simulink model "Base_Map_S_P_L_cs"  (R2019a)
settings: Solver=FixedStepDiscrete  StartTime=0.0  StopTime=inf  FixedStep=1/300  RelTol=1e-3
PreLoadFcn:
  | mbxruntime.callbacks.PreLoadFcn(bdroot);
  | check_NUTS_defined
  | model_closed = 0;
  | assignin('base',['model_closed_' bdroot],false);
PostLoadFcn:
  | mbxruntime.callbacks.PostLoadFcn(bdroot);
InitFcn:
  | mbxruntime.callbacks.InitFcn(bdroot);
StartFcn:
  | mbxruntime.callbacks.StartFcn(bdroot);
StopFcn:
  | mbxruntime.callbacks.StopFcn(bdroot);;
  | 
model workspace: external: MAT-File .\Base_Map_S_P_L_cs_hws.mat (data not in the file)
undefined symbols (not defined in the file): DiscIntNeverNeededParam, Header, InitImageOutputDir, mbxruntime, Orientation, Pose, Poses, Poses_SL_Info, Position, tabledata
libraries: PBCSimulinkLibrary x53, simulink_extras x9, PreScanSimulinkLibrary x6, robotlib x6, PreScanUsefulBlocks x4, sharedtransform x3, aerolibutil x2, visionconversions x1, visionsinks x1
(part 5 of 7)

== system Base_Map_S_P_L_cs/Citroen_C3_Hatchback_1/Car_Pos_and_Orient ==
  In1 : Inport
  In2 : Inport  Port=2
  In3 : Inport  Port=3
  In4 : Inport  Port=4
  In5 : Inport  Port=5
  In6 : Inport  Port=6
  Data Type Conversion : DataTypeConversion
  Data Type Conversion1 : DataTypeConversion
  Data Type Conversion2 : DataTypeConversion
  Degrees to Radians1 : simulink_extras/Transformations/Degrees to Radians
  Degrees to Radians2 : simulink_extras/Transformations/Degrees to Radians
  Degrees to Radians5 : simulink_extras/Transformations/Degrees to Radians
  Mux : Mux
  Rotation Angles to Quaternions : sharedtransform/Rotation Angles to Quaternions  rotationOrder=XYZ  aMode=aMode
      settings: SourceProductName=Aerospace Blockset  SourceProductBaseCode=AE
  Vector Concatenate2 : Concatenate  NumInputs=3
  Out1 : Outport
  wires:
  Degrees to Radians1/1 -> Vector Concatenate2/2
  Degrees to Radians5/1 -> Vector Concatenate2/1
  Vector Concatenate2/1 -> Rotation Angles to Quaternions/1
  Degrees to Radians2/1 -> Vector Concatenate2/3
  In1/1 -> Data Type Conversion/1
  In2/1 -> Data Type Conversion1/1
  In3/1 -> Data Type Conversion2/1
  In4/1 -> Degrees to Radians5/1
  In5/1 -> Degrees to Radians1/1
  In6/1 -> Degrees to Radians2/1
  Data Type Conversion/1 -> Mux/1
  Data Type Conversion1/1 -> Mux/2
  Data Type Conversion2/1 -> Mux/3
  Rotation Angles to Quaternions/1 -> Mux/4
  Mux/1 -> Out1/1

== system Base_Map_S_P_L_cs/Citroen_C3_Hatchback_1/Dynamics_Empty ==
  note: For state mode 'Dynamic' positions
      | are not taken into account, as they
      | are computed by integrating velocity.
      | Click annotation for Help.
  Ground_{1..8} (8 alike) : Ground
  MuxState : Subsystem  Tag=mux/State  mask(Empty Dynamics State Block){positioningmode=on, TimeStep=1/300}
      mask prompts: positioningmode "Positioning Mode"; TimeStep "Auto Assigned: Time Step [s]"
      mask help:
      | Build the state of an actor based on user input.
      | The user can either use positioning mode or dynamics mode.
      | - When using positioning mode the position and orientation of the actor are set directly based on the input. Expected input is relative to the initial position and orientation of the actor. It's also possible to specify the velocity of the actor, though this input isn't used, only passed on.
      | - When using dynamics mode the position input is ignored. Expected input is velocity and orientation. The velocity is relative the current orientation of the actor, while orientation is relative to its initial orientation. The position of the actor is calculated based on the velocity and orientation given.
      settings: DeleteFcn=PreScanBlockDeleteFcn;
  STATE_Citroen_C3_Hatchback_1 : Subsystem  Tag=mux/StatePort  Priority=0  LoadFcn=load PrescanStateActuatorData  mask(PreScan Sink Block: State){x0=181.3426, y0=102.1129, z0=0.58, Roll0=0, Pitch0=0, Yaw0=0, TimeStep=1/300}
      mask prompts: x0 "Ini x-position VEHICLE wrt GLOBAL axis system [m]"; y0 "Ini y-position VEHICLE wrt GLOBAL axis system [m]"; z0 "Ini z-position VEHICLE wrt GLOBAL axis system [m]"; Roll0 "Ini roll-angle BODY wrt VEHICLE axis system [deg]"; Pitch0 "Ini pitch-angle BODY wrt VEHICLE axis system [deg]"; Yaw0 "Ini yaw-angle VEHICLE wrt GLOBAL axis system [deg]"; TimeStep "Auto-Assigned: Upload Period [s]"
      mask help:
      | The Actor State contains a vector signal of size (9x1), containing the following signals:
      |
      | -  Position                  (x,y,z)                                     [m]
      | -  Velocity                  (vx,vy,vz)                               [m/s]
      | -  Angles                    (Roll, Pitch, Yaw)                   [rad]
      |
      | The Actor state is defined in the global axis system.
      | The state is superponed on the Initial position defined in the GUI.
      |
      | For more information, please click Help.
      settings: DeleteFcn=PreScanBlockDeleteFcn;
      mask Help: eval('openHelp(222)')
      mask Display: image(imread('State.png'))
  Sine Wave Function : Sin  Amplitude=10  SampleTime=0
  State : Outport  Tag=outport/StateOutport  SampleTime=1/300
  wires:
  Sine Wave Function/1 -> MuxState/1(x [m])
  MuxState/1(state) -> STATE_Citroen_C3_Hatchback_1/1(State)
  STATE_Citroen_C3_Hatchback_1/1(StateBus) -> State/1
  Ground_1/1 -> MuxState/2(y [m])
  Ground_2/1 -> MuxState/3(z [m])
  Ground_3/1 -> MuxState/4(dx [m/s])
  Ground_4/1 -> MuxState/5(dy [m/s])
  Ground_5/1 -> MuxState/6(dz [m/s])
  Ground_6/1 -> MuxState/7(R [rad])
  Ground_7/1 -> MuxState/8(P [rad])
  Ground_8/1 -> MuxState/9(Y [rad])

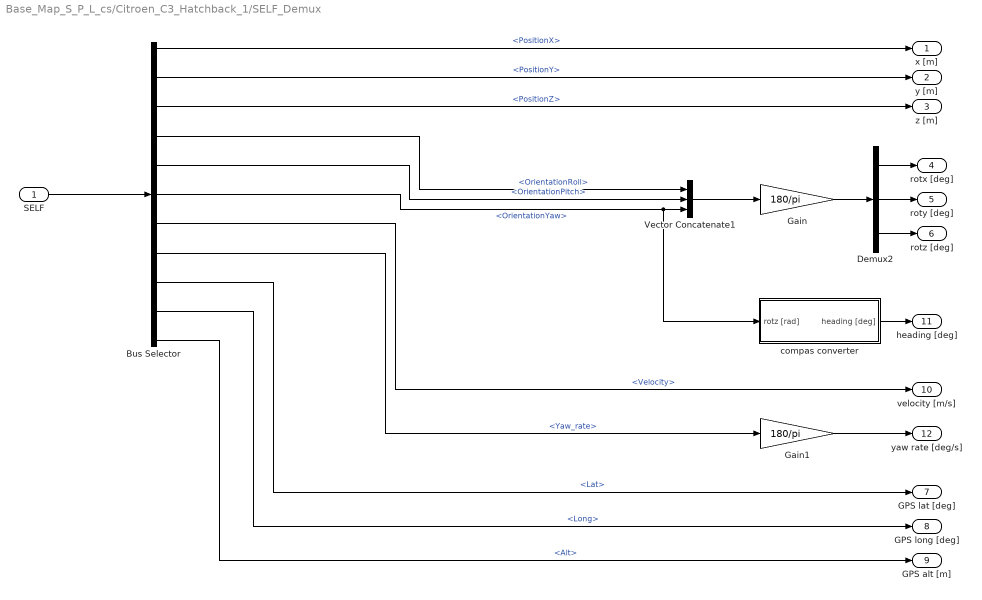
== system Base_Map_S_P_L_cs/Citroen_C3_Hatchback_1/SELF_Demux ==
  SELF : Inport  OutDataTypeStr=Bus: PRESCAN_SELFSENSORDATA
  Bus Selector : BusSelector  OutputSignals=PositionX,PositionY,PositionZ,OrientationRoll,OrientationPitch,OrientationYaw,Velocity,Yaw_rate,Lat,Long,Alt
  Demux2 : Demux  Outputs=3
  Gain : Gain  Gain=180/pi
  Gain1 : Gain  Gain=180/pi
  Vector Concatenate1 : Concatenate  NumInputs=3
  compas converter : Subsystem
  x [m] : Outport
  y [m] : Outport  Port=2
  z [m] : Outport  Port=3
  rotx [deg] : Outport  Port=4
  roty [deg] : Outport  Port=5
  rotz [deg] : Outport  Port=6
  GPS lat [deg] : Outport  Port=7
  GPS long [deg] : Outport  Port=8
  GPS alt [m] : Outport  Port=9
  velocity [m/s] : Outport  Port=10
  heading [deg] : Outport  Port=11
  yaw rate [deg/s] : Outport  Port=12
  wires:
  Bus Selector/11 -> GPS alt [m]/1  "<Alt>"
  Bus Selector/10 -> GPS long [deg]/1  "<Long>"
  Bus Selector/9 -> GPS lat [deg]/1  "<Lat>"
  Bus Selector/8 -> Gain1/1  "<Yaw_rate>"
  Bus Selector/7 -> velocity [m/s]/1  "<Velocity>"
  Bus Selector/6 -> compas converter/1(rotz [rad]), Vector Concatenate1/3  "<OrientationYaw>"
  Bus Selector/5 -> Vector Concatenate1/2  "<OrientationPitch>"
  Bus Selector/4 -> Vector Concatenate1/1  "<OrientationRoll>"
  Vector Concatenate1/1 -> Gain/1
  Bus Selector/3 -> z [m]/1  "<PositionZ>"
  Bus Selector/2 -> y [m]/1  "<PositionY>"
  Bus Selector/1 -> x [m]/1  "<PositionX>"
  SELF/1 -> Bus Selector/1
  Gain/1 -> Demux2/1
  Demux2/1 -> rotx [deg]/1
  Demux2/2 -> roty [deg]/1
  Demux2/3 -> rotz [deg]/1
  compas converter/1(heading [deg]) -> heading [deg]/1
  Gain1/1 -> yaw rate [deg/s]/1

== system Base_Map_S_P_L_cs/Citroen_C3_Hatchback_1/message_creator ==
  In1 : Inport
  Blank Message4 : robotlib/Blank Message  messageClass=Message  entityType=geometry_msgs/Pose  messageType=geometry_msgs/Pose  SampleTime=inf
      settings: SourceProductBaseCode=RO
  Bus Assignment3 : BusAssignment  AssignedSignals=Position.X,Position.Y,Position.Z,Orientation.W,Orientation.X,Orientation.Y,Orientation.Z
  Demux : Demux  Outputs=7
  Out1 : Outport
  wires:
  Blank Message4/1 -> Bus Assignment3/1
  Demux/4 -> Bus Assignment3/5
  Demux/3 -> Bus Assignment3/4
  Demux/5 -> Bus Assignment3/6
  Demux/7 -> Bus Assignment3/8
  Demux/2 -> Bus Assignment3/3
  In1/1 -> Demux/1
  Demux/6 -> Bus Assignment3/7
  Demux/1 -> Bus Assignment3/2
  Bus Assignment3/1 -> Out1/1

== system Base_Map_S_P_L_cs/Ford_Fiesta_Hatchback_1/AIR_1_Demux ==
  AIR : Inport
  Activate_Switch : Subsystem
      mask Display: text(5,10,'')
  Bus Selector : BusSelector  OutputSignals=DATA.Range,DATA.Azimuth,DATA.Elevation,DATA.ID,DATA.Velocity,DATA.Heading
  Data Type Conversion : DataTypeConversion  OutDataTypeStr=double
  For Iterator : ForIterator  ResetStates=reset  IterationLimit=detectableObjects
  Selector : Selector  InputPortWidth=detectableObjects  IndexOptions=Index vector (port)  Indices=[1 3]  OutputSizes=1
  Signal2ArrayOfSignals1 : Subsystem  mask{VECTORLENGTH=detectableObjects}
      mask prompts: VECTORLENGTH "Length of vector"
  Signal2ArrayOfSignals2 : Subsystem  mask{VECTORLENGTH=detectableObjects}
      mask prompts: VECTORLENGTH "Length of vector"
  Signal2ArrayOfSignals3 : Subsystem  mask{VECTORLENGTH=detectableObjects}
      mask prompts: VECTORLENGTH "Length of vector"
  Signal2ArrayOfSignals4 : Subsystem  mask{VECTORLENGTH=detectableObjects}
      mask prompts: VECTORLENGTH "Length of vector"
  Signal2ArrayOfSignals5 : Subsystem  mask{VECTORLENGTH=detectableObjects}
      mask prompts: VECTORLENGTH "Length of vector"
  Signal2ArrayOfSignals6 : Subsystem  mask{VECTORLENGTH=detectableObjects}
      mask prompts: VECTORLENGTH "Length of vector"
  Range [m] : Outport
  Azimuth [deg] : Outport  Port=2
  Elevation [deg] : Outport  Port=3
  ID [-] : Outport  Port=4
  Velocity [m/s] : Outport  Port=5
  Heading [deg] : Outport  Port=6
  wires:
  Data Type Conversion/1 -> ID [-]/1
  Bus Selector/6 -> Signal2ArrayOfSignals6/2(Element)  "<Heading>"
  Signal2ArrayOfSignals6/1(ArrayofElements) -> Activate_Switch/2(Heading)
  Bus Selector/5 -> Signal2ArrayOfSignals5/2(Element)  "<Velocity>"
  Signal2ArrayOfSignals5/1(ArrayofElements) -> Velocity [m/s]/1
  Bus Selector/4 -> Signal2ArrayOfSignals4/2(Element)  "<ID>"
  Signal2ArrayOfSignals4/1(ArrayofElements) -> Data Type Conversion/1, Activate_Switch/1(BeamID)
  Bus Selector/3 -> Signal2ArrayOfSignals3/2(Element)  "<Elevation>"
  Signal2ArrayOfSignals3/1(ArrayofElements) -> Elevation [deg]/1
  Bus Selector/2 -> Signal2ArrayOfSignals1/2(Element)  "<Azimuth>"
  Signal2ArrayOfSignals1/1(ArrayofElements) -> Azimuth [deg]/1
  Signal2ArrayOfSignals2/1(ArrayofElements) -> Range [m]/1
  Bus Selector/1 -> Signal2ArrayOfSignals2/2(Element)  "<Range>"
  Selector/1 -> Bus Selector/1
  For Iterator/1 -> Signal2ArrayOfSignals6/1(LoopIndex), Signal2ArrayOfSignals5/1(LoopIndex), Signal2ArrayOfSignals4/1(LoopIndex), Signal2ArrayOfSignals3/1(LoopIndex), Signal2ArrayOfSignals1/1(LoopIndex), Signal2ArrayOfSignals2/1(LoopIndex), Selector/2
  AIR/1 -> Selector/1
  Activate_Switch/1(On/Off) -> Heading [deg]/1

== system Base_Map_S_P_L_cs/Ford_Fiesta_Hatchback_1/Car_Pos_and_Orient ==
  In1 : Inport
  In2 : Inport  Port=2
  In3 : Inport  Port=3
  In4 : Inport  Port=4
  In5 : Inport  Port=5
  In6 : Inport  Port=6
  Data Type Conversion : DataTypeConversion
  Data Type Conversion1 : DataTypeConversion
  Data Type Conversion2 : DataTypeConversion
  Degrees to Radians1 : simulink_extras/Transformations/Degrees to Radians
  Degrees to Radians2 : simulink_extras/Transformations/Degrees to Radians
  Degrees to Radians5 : simulink_extras/Transformations/Degrees to Radians
  Mux : Mux
  Rotation Angles to Quaternions : sharedtransform/Rotation Angles to Quaternions  rotationOrder=XYZ  aMode=aMode
      settings: SourceProductName=Aerospace Blockset  SourceProductBaseCode=AE
  Vector Concatenate2 : Concatenate  NumInputs=3
  Out1 : Outport
  wires:
  Degrees to Radians1/1 -> Vector Concatenate2/2
  Degrees to Radians5/1 -> Vector Concatenate2/1
  Vector Concatenate2/1 -> Rotation Angles to Quaternions/1
  Degrees to Radians2/1 -> Vector Concatenate2/3
  In1/1 -> Data Type Conversion/1
  In2/1 -> Data Type Conversion1/1
  In3/1 -> Data Type Conversion2/1
  In4/1 -> Degrees to Radians5/1
  In5/1 -> Degrees to Radians1/1
  In6/1 -> Degrees to Radians2/1
  Data Type Conversion/1 -> Mux/1
  Data Type Conversion1/1 -> Mux/2
  Data Type Conversion2/1 -> Mux/3
  Rotation Angles to Quaternions/1 -> Mux/4
  Mux/1 -> Out1/1

== system Base_Map_S_P_L_cs/Ford_Fiesta_Hatchback_1/Dynamics_Empty ==
  note: For state mode 'Dynamic' positions
      | are not taken into account, as they
      | are computed by integrating velocity.
      | Click annotation for Help.
  Ground_{1..9} (9 alike) : Ground
  MuxState : Subsystem  Tag=mux/State  mask(Empty Dynamics State Block){positioningmode=on, TimeStep=1/300}
      mask prompts: positioningmode "Positioning Mode"; TimeStep "Auto Assigned: Time Step [s]"
      mask help:
      | Build the state of an actor based on user input.
      | The user can either use positioning mode or dynamics mode.
      | - When using positioning mode the position and orientation of the actor are set directly based on the input. Expected input is relative to the initial position and orientation of the actor. It's also possible to specify the velocity of the actor, though this input isn't used, only passed on.
      | - When using dynamics mode the position input is ignored. Expected input is velocity and orientation. The velocity is relative the current orientation of the actor, while orientation is relative to its initial orientation. The position of the actor is calculated based on the velocity and orientation given.
      settings: DeleteFcn=PreScanBlockDeleteFcn;
  STATE_Ford_Fiesta_Hatchback_1 : Subsystem  Tag=mux/StatePort  Priority=0  LoadFcn=load PrescanStateActuatorData  mask(PreScan Sink Block: State){x0=127.763, y0=175.1293, z0=0.53, Roll0=0, Pitch0=0, Yaw0=1.7357, TimeStep=1/300}
      mask prompts: x0 "Ini x-position VEHICLE wrt GLOBAL axis system [m]"; y0 "Ini y-position VEHICLE wrt GLOBAL axis system [m]"; z0 "Ini z-position VEHICLE wrt GLOBAL axis system [m]"; Roll0 "Ini roll-angle BODY wrt VEHICLE axis system [deg]"; Pitch0 "Ini pitch-angle BODY wrt VEHICLE axis system [deg]"; Yaw0 "Ini yaw-angle VEHICLE wrt GLOBAL axis system [deg]"; TimeStep "Auto-Assigned: Upload Period [s]"
      mask help:
      | The Actor State contains a vector signal of size (9x1), containing the following signals:
      |
      | -  Position                  (x,y,z)                                     [m]
      | -  Velocity                  (vx,vy,vz)                               [m/s]
      | -  Angles                    (Roll, Pitch, Yaw)                   [rad]
      |
      | The Actor state is defined in the global axis system.
      | The state is superponed on the Initial position defined in the GUI.
      |
      | For more information, please click Help.
      settings: DeleteFcn=PreScanBlockDeleteFcn;
      mask Help: eval('openHelp(222)')
      mask Display: image(imread('State.png'))
  State : Outport  Tag=outport/StateOutport  SampleTime=1/300
  wires:
  MuxState/1(state) -> STATE_Ford_Fiesta_Hatchback_1/1(State)
  STATE_Ford_Fiesta_Hatchback_1/1(StateBus) -> State/1
  Ground_1/1 -> MuxState/1(x [m])
  Ground_2/1 -> MuxState/2(y [m])
  Ground_3/1 -> MuxState/3(z [m])
  Ground_4/1 -> MuxState/4(dx [m/s])
  Ground_5/1 -> MuxState/5(dy [m/s])
  Ground_6/1 -> MuxState/6(dz [m/s])
  Ground_7/1 -> MuxState/7(R [rad])
  Ground_8/1 -> MuxState/8(P [rad])
  Ground_9/1 -> MuxState/9(Y [rad])

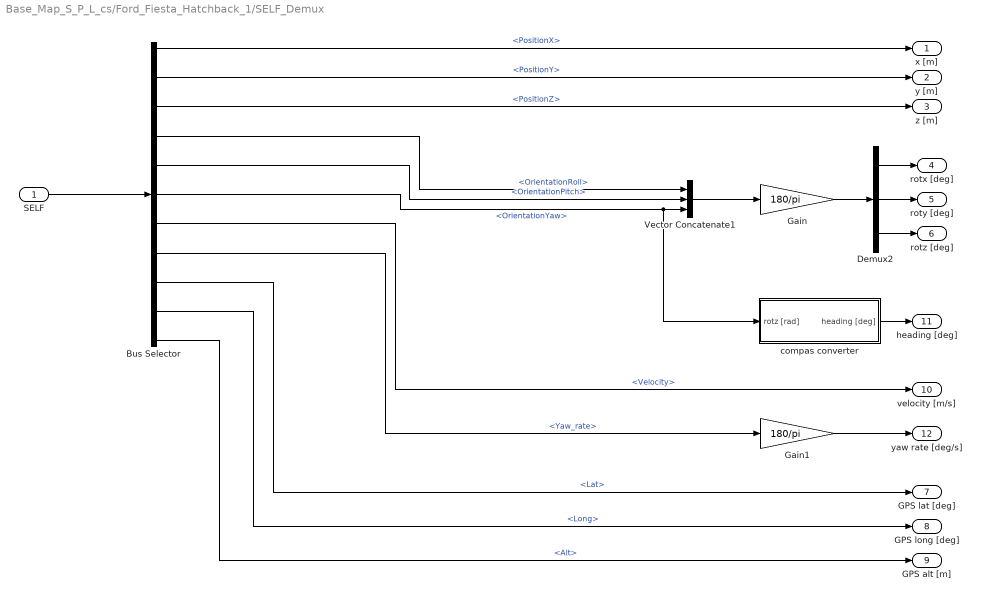
== system Base_Map_S_P_L_cs/Ford_Fiesta_Hatchback_1/SELF_Demux ==
  SELF : Inport  OutDataTypeStr=Bus: PRESCAN_SELFSENSORDATA
  Bus Selector : BusSelector  OutputSignals=PositionX,PositionY,PositionZ,OrientationRoll,OrientationPitch,OrientationYaw,Velocity,Yaw_rate,Lat,Long,Alt
  Demux2 : Demux  Outputs=3
  Gain : Gain  Gain=180/pi
  Gain1 : Gain  Gain=180/pi
  Vector Concatenate1 : Concatenate  NumInputs=3
  compas converter : Subsystem
  x [m] : Outport
  y [m] : Outport  Port=2
  z [m] : Outport  Port=3
  rotx [deg] : Outport  Port=4
  roty [deg] : Outport  Port=5
  rotz [deg] : Outport  Port=6
  GPS lat [deg] : Outport  Port=7
  GPS long [deg] : Outport  Port=8
  GPS alt [m] : Outport  Port=9
  velocity [m/s] : Outport  Port=10
  heading [deg] : Outport  Port=11
  yaw rate [deg/s] : Outport  Port=12
  wires:
  Bus Selector/11 -> GPS alt [m]/1  "<Alt>"
  Bus Selector/10 -> GPS long [deg]/1  "<Long>"
  Bus Selector/9 -> GPS lat [deg]/1  "<Lat>"
  Bus Selector/8 -> Gain1/1  "<Yaw_rate>"
  Bus Selector/7 -> velocity [m/s]/1  "<Velocity>"
  Bus Selector/6 -> compas converter/1(rotz [rad]), Vector Concatenate1/3  "<OrientationYaw>"
  Bus Selector/5 -> Vector Concatenate1/2  "<OrientationPitch>"
  Bus Selector/4 -> Vector Concatenate1/1  "<OrientationRoll>"
  Vector Concatenate1/1 -> Gain/1
  Bus Selector/3 -> z [m]/1  "<PositionZ>"
  Bus Selector/2 -> y [m]/1  "<PositionY>"
  Bus Selector/1 -> x [m]/1  "<PositionX>"
  SELF/1 -> Bus Selector/1
  Gain/1 -> Demux2/1
  Demux2/1 -> rotx [deg]/1
  Demux2/2 -> roty [deg]/1
  Demux2/3 -> rotz [deg]/1
  compas converter/1(heading [deg]) -> heading [deg]/1
  Gain1/1 -> yaw rate [deg/s]/1

== system Base_Map_S_P_L_cs/Ford_Fiesta_Hatchback_1/message_creator ==
  In1 : Inport
  Blank Message4 : robotlib/Blank Message  messageClass=Message  entityType=geometry_msgs/Pose  messageType=geometry_msgs/Pose  SampleTime=inf
      settings: SourceProductBaseCode=RO
  Bus Assignment3 : BusAssignment  AssignedSignals=Position.X,Position.Y,Position.Z,Orientation.W,Orientation.X,Orientation.Y,Orientation.Z
  Demux : Demux  Outputs=7
  Out1 : Outport
  wires:
  Blank Message4/1 -> Bus Assignment3/1
  Demux/4 -> Bus Assignment3/5
  Demux/3 -> Bus Assignment3/4
  Demux/5 -> Bus Assignment3/6
  Demux/7 -> Bus Assignment3/8
  Demux/2 -> Bus Assignment3/3
  In1/1 -> Demux/1
  Demux/6 -> Bus Assignment3/7
  Demux/1 -> Bus Assignment3/2
  Bus Assignment3/1 -> Out1/1

== system Base_Map_S_P_L_cs/TrafficLightRoadSideNL_1/TrafficLightRoadSideNL_1_Casing.LightGreen_Control_Mux ==
  SPDIndex [-] : Inport
  Power [W] : Inport  Port=2
  Bus Creator1 : BusCreator  Inputs=4  OutDataTypeStr=Bus: PRESCAN_PBCLIGHT_DATA  NonVirtualBus=on
  Double2Uint : DataTypeConversion  OutDataTypeStr=uint32
  NonNegativeSignalChanged1 : PBCSimulinkLibrary/NonNegativeSignalChanged  SystemSampleTime=-1
  NonNegativeSignalChanged2 : PBCSimulinkLibrary/NonNegativeSignalChanged  SystemSampleTime=-1
  Bus : Outport
  wires:
  Double2Uint/1 -> Bus Creator1/2  "SPDIndex"
  NonNegativeSignalChanged2/1 -> Bus Creator1/3  "PowerDefined"
  NonNegativeSignalChanged1/1 -> Bus Creator1/1  "SPDIndexDefined"
  Power [W]/1 -> Bus Creator1/4, NonNegativeSignalChanged2/1  "Power"
  SPDIndex [-]/1 -> Double2Uint/1, NonNegativeSignalChanged1/1  "SPDIndex"
  Bus Creator1/1 -> Bus/1

== system Base_Map_S_P_L_cs/TrafficLightRoadSideNL_1/TrafficLightRoadSideNL_1_Casing.LightOrange_Control_Mux ==
  SPDIndex [-] : Inport
  Power [W] : Inport  Port=2
  Bus Creator1 : BusCreator  Inputs=4  OutDataTypeStr=Bus: PRESCAN_PBCLIGHT_DATA  NonVirtualBus=on
  Double2Uint : DataTypeConversion  OutDataTypeStr=uint32
  NonNegativeSignalChanged1 : PBCSimulinkLibrary/NonNegativeSignalChanged  SystemSampleTime=-1
  NonNegativeSignalChanged2 : PBCSimulinkLibrary/NonNegativeSignalChanged  SystemSampleTime=-1
  Bus : Outport
  wires:
  Double2Uint/1 -> Bus Creator1/2  "SPDIndex"
  NonNegativeSignalChanged2/1 -> Bus Creator1/3  "PowerDefined"
  NonNegativeSignalChanged1/1 -> Bus Creator1/1  "SPDIndexDefined"
  Power [W]/1 -> Bus Creator1/4, NonNegativeSignalChanged2/1  "Power"
  SPDIndex [-]/1 -> Double2Uint/1, NonNegativeSignalChanged1/1  "SPDIndex"
  Bus Creator1/1 -> Bus/1

== system Base_Map_S_P_L_cs/TrafficLightRoadSideNL_1/TrafficLightRoadSideNL_1_Casing.LightRed_Control_Mux ==
  SPDIndex [-] : Inport
  Power [W] : Inport  Port=2
  Bus Creator1 : BusCreator  Inputs=4  OutDataTypeStr=Bus: PRESCAN_PBCLIGHT_DATA  NonVirtualBus=on
  Double2Uint : DataTypeConversion  OutDataTypeStr=uint32
  NonNegativeSignalChanged1 : PBCSimulinkLibrary/NonNegativeSignalChanged  SystemSampleTime=-1
  NonNegativeSignalChanged2 : PBCSimulinkLibrary/NonNegativeSignalChanged  SystemSampleTime=-1
  Bus : Outport
  wires:
  Double2Uint/1 -> Bus Creator1/2  "SPDIndex"
  NonNegativeSignalChanged2/1 -> Bus Creator1/3  "PowerDefined"
  NonNegativeSignalChanged1/1 -> Bus Creator1/1  "SPDIndexDefined"
  Power [W]/1 -> Bus Creator1/4, NonNegativeSignalChanged2/1  "Power"
  SPDIndex [-]/1 -> Double2Uint/1, NonNegativeSignalChanged1/1  "SPDIndex"
  Bus Creator1/1 -> Bus/1

== system Base_Map_S_P_L_cs/TrafficLightRoadSideNL_1/VISUCasingLights_Mux ==
  Green [-] : Inport  Tag=inport/Green [-]  SampleTime=1/300  BusOutputAsStruct=on
  Orange [-] : Inport  Tag=inport/Orange [-]  Port=2  SampleTime=1/300  BusOutputAsStruct=on
  Red [-] : Inport  Tag=inport/Red [-]  Port=3  SampleTime=1/300  BusOutputAsStruct=on
  MuxVisuLights : Mux  Inputs=3
  VISUCasingLights_TrafficLightRoadSideNL_1 : Outport  Tag=outport/VisuCasingLights  SampleTime=1/300
  wires:
  MuxVisuLights/1 -> VISUCasingLights_TrafficLightRoadSideNL_1/1
  Green [-]/1 -> MuxVisuLights/1
  Orange [-]/1 -> MuxVisuLights/2
  Red [-]/1 -> MuxVisuLights/3

== system Base_Map_S_P_L_cs/TrafficLightRoadSideNL_2/TrafficLightRoadSideNL_2_Casing.LightGreen_Control_Mux ==
  SPDIndex [-] : Inport
  Power [W] : Inport  Port=2
  Bus Creator1 : BusCreator  Inputs=4  OutDataTypeStr=Bus: PRESCAN_PBCLIGHT_DATA  NonVirtualBus=on
  Double2Uint : DataTypeConversion  OutDataTypeStr=uint32
  NonNegativeSignalChanged1 : PBCSimulinkLibrary/NonNegativeSignalChanged  SystemSampleTime=-1
  NonNegativeSignalChanged2 : PBCSimulinkLibrary/NonNegativeSignalChanged  SystemSampleTime=-1
  Bus : Outport
  wires:
  Double2Uint/1 -> Bus Creator1/2  "SPDIndex"
  NonNegativeSignalChanged2/1 -> Bus Creator1/3  "PowerDefined"
  NonNegativeSignalChanged1/1 -> Bus Creator1/1  "SPDIndexDefined"
  Power [W]/1 -> Bus Creator1/4, NonNegativeSignalChanged2/1  "Power"
  SPDIndex [-]/1 -> Double2Uint/1, NonNegativeSignalChanged1/1  "SPDIndex"
  Bus Creator1/1 -> Bus/1

== system Base_Map_S_P_L_cs/TrafficLightRoadSideNL_2/TrafficLightRoadSideNL_2_Casing.LightOrange_Control_Mux ==
  SPDIndex [-] : Inport
  Power [W] : Inport  Port=2
  Bus Creator1 : BusCreator  Inputs=4  OutDataTypeStr=Bus: PRESCAN_PBCLIGHT_DATA  NonVirtualBus=on
  Double2Uint : DataTypeConversion  OutDataTypeStr=uint32
  NonNegativeSignalChanged1 : PBCSimulinkLibrary/NonNegativeSignalChanged  SystemSampleTime=-1
  NonNegativeSignalChanged2 : PBCSimulinkLibrary/NonNegativeSignalChanged  SystemSampleTime=-1
  Bus : Outport
  wires:
  Double2Uint/1 -> Bus Creator1/2  "SPDIndex"
  NonNegativeSignalChanged2/1 -> Bus Creator1/3  "PowerDefined"
  NonNegativeSignalChanged1/1 -> Bus Creator1/1  "SPDIndexDefined"
  Power [W]/1 -> Bus Creator1/4, NonNegativeSignalChanged2/1  "Power"
  SPDIndex [-]/1 -> Double2Uint/1, NonNegativeSignalChanged1/1  "SPDIndex"
  Bus Creator1/1 -> Bus/1

== system Base_Map_S_P_L_cs/TrafficLightRoadSideNL_2/TrafficLightRoadSideNL_2_Casing.LightRed_Control_Mux ==
  SPDIndex [-] : Inport
  Power [W] : Inport  Port=2
  Bus Creator1 : BusCreator  Inputs=4  OutDataTypeStr=Bus: PRESCAN_PBCLIGHT_DATA  NonVirtualBus=on
  Double2Uint : DataTypeConversion  OutDataTypeStr=uint32
  NonNegativeSignalChanged1 : PBCSimulinkLibrary/NonNegativeSignalChanged  SystemSampleTime=-1
  NonNegativeSignalChanged2 : PBCSimulinkLibrary/NonNegativeSignalChanged  SystemSampleTime=-1
  Bus : Outport
  wires:
  Double2Uint/1 -> Bus Creator1/2  "SPDIndex"
  NonNegativeSignalChanged2/1 -> Bus Creator1/3  "PowerDefined"
  NonNegativeSignalChanged1/1 -> Bus Creator1/1  "SPDIndexDefined"
  Power [W]/1 -> Bus Creator1/4, NonNegativeSignalChanged2/1  "Power"
  SPDIndex [-]/1 -> Double2Uint/1, NonNegativeSignalChanged1/1  "SPDIndex"
  Bus Creator1/1 -> Bus/1

== system Base_Map_S_P_L_cs/TrafficLightRoadSideNL_2/VISUCasingLights_Mux ==
  Green [-] : Inport  Tag=inport/Green [-]  SampleTime=1/300  BusOutputAsStruct=on
  Orange [-] : Inport  Tag=inport/Orange [-]  Port=2  SampleTime=1/300  BusOutputAsStruct=on
  Red [-] : Inport  Tag=inport/Red [-]  Port=3  SampleTime=1/300  BusOutputAsStruct=on
  MuxVisuLights : Mux  Inputs=3
  VISUCasingLights_TrafficLightRoadSideNL_2 : Outport  Tag=outport/VisuCasingLights  SampleTime=1/300
  wires:
  MuxVisuLights/1 -> VISUCasingLights_TrafficLightRoadSideNL_2/1
  Green [-]/1 -> MuxVisuLights/1
  Orange [-]/1 -> MuxVisuLights/2
  Red [-]/1 -> MuxVisuLights/3

== system Base_Map_S_P_L_cs/TrafficLightRoadSideNL_3/TrafficLightRoadSideNL_3_Casing.LightGreen_Control_Mux ==
  SPDIndex [-] : Inport
  Power [W] : Inport  Port=2
  Bus Creator1 : BusCreator  Inputs=4  OutDataTypeStr=Bus: PRESCAN_PBCLIGHT_DATA  NonVirtualBus=on
  Double2Uint : DataTypeConversion  OutDataTypeStr=uint32
  NonNegativeSignalChanged1 : PBCSimulinkLibrary/NonNegativeSignalChanged  SystemSampleTime=-1
  NonNegativeSignalChanged2 : PBCSimulinkLibrary/NonNegativeSignalChanged  SystemSampleTime=-1
  Bus : Outport
  wires:
  Double2Uint/1 -> Bus Creator1/2  "SPDIndex"
  NonNegativeSignalChanged2/1 -> Bus Creator1/3  "PowerDefined"
  NonNegativeSignalChanged1/1 -> Bus Creator1/1  "SPDIndexDefined"
  Power [W]/1 -> Bus Creator1/4, NonNegativeSignalChanged2/1  "Power"
  SPDIndex [-]/1 -> Double2Uint/1, NonNegativeSignalChanged1/1  "SPDIndex"
  Bus Creator1/1 -> Bus/1

== system Base_Map_S_P_L_cs/TrafficLightRoadSideNL_3/TrafficLightRoadSideNL_3_Casing.LightOrange_Control_Mux ==
  SPDIndex [-] : Inport
  Power [W] : Inport  Port=2
  Bus Creator1 : BusCreator  Inputs=4  OutDataTypeStr=Bus: PRESCAN_PBCLIGHT_DATA  NonVirtualBus=on
  Double2Uint : DataTypeConversion  OutDataTypeStr=uint32
  NonNegativeSignalChanged1 : PBCSimulinkLibrary/NonNegativeSignalChanged  SystemSampleTime=-1
  NonNegativeSignalChanged2 : PBCSimulinkLibrary/NonNegativeSignalChanged  SystemSampleTime=-1
  Bus : Outport
  wires:
  Double2Uint/1 -> Bus Creator1/2  "SPDIndex"
  NonNegativeSignalChanged2/1 -> Bus Creator1/3  "PowerDefined"
  NonNegativeSignalChanged1/1 -> Bus Creator1/1  "SPDIndexDefined"
  Power [W]/1 -> Bus Creator1/4, NonNegativeSignalChanged2/1  "Power"
  SPDIndex [-]/1 -> Double2Uint/1, NonNegativeSignalChanged1/1  "SPDIndex"
  Bus Creator1/1 -> Bus/1

== system Base_Map_S_P_L_cs/TrafficLightRoadSideNL_3/TrafficLightRoadSideNL_3_Casing.LightRed_Control_Mux ==
  SPDIndex [-] : Inport
  Power [W] : Inport  Port=2
  Bus Creator1 : BusCreator  Inputs=4  OutDataTypeStr=Bus: PRESCAN_PBCLIGHT_DATA  NonVirtualBus=on
  Double2Uint : DataTypeConversion  OutDataTypeStr=uint32
  NonNegativeSignalChanged1 : PBCSimulinkLibrary/NonNegativeSignalChanged  SystemSampleTime=-1
  NonNegativeSignalChanged2 : PBCSimulinkLibrary/NonNegativeSignalChanged  SystemSampleTime=-1
  Bus : Outport
  wires:
  Double2Uint/1 -> Bus Creator1/2  "SPDIndex"
  NonNegativeSignalChanged2/1 -> Bus Creator1/3  "PowerDefined"
  NonNegativeSignalChanged1/1 -> Bus Creator1/1  "SPDIndexDefined"
  Power [W]/1 -> Bus Creator1/4, NonNegativeSignalChanged2/1  "Power"
  SPDIndex [-]/1 -> Double2Uint/1, NonNegativeSignalChanged1/1  "SPDIndex"
  Bus Creator1/1 -> Bus/1

== system Base_Map_S_P_L_cs/TrafficLightRoadSideNL_3/VISUCasingLights_Mux ==
  Green [-] : Inport  Tag=inport/Green [-]  SampleTime=1/300  BusOutputAsStruct=on
  Orange [-] : Inport  Tag=inport/Orange [-]  Port=2  SampleTime=1/300  BusOutputAsStruct=on
  Red [-] : Inport  Tag=inport/Red [-]  Port=3  SampleTime=1/300  BusOutputAsStruct=on
  MuxVisuLights : Mux  Inputs=3
  VISUCasingLights_TrafficLightRoadSideNL_3 : Outport  Tag=outport/VisuCasingLights  SampleTime=1/300
  wires:
  MuxVisuLights/1 -> VISUCasingLights_TrafficLightRoadSideNL_3/1
  Green [-]/1 -> MuxVisuLights/1
  Orange [-]/1 -> MuxVisuLights/2
  Red [-]/1 -> MuxVisuLights/3

== system Base_Map_S_P_L_cs/TrafficLightRoadSideNL_4/TrafficLightRoadSideNL_4_Casing.LightGreen_Control_Mux ==
  SPDIndex [-] : Inport
  Power [W] : Inport  Port=2
  Bus Creator1 : BusCreator  Inputs=4  OutDataTypeStr=Bus: PRESCAN_PBCLIGHT_DATA  NonVirtualBus=on
  Double2Uint : DataTypeConversion  OutDataTypeStr=uint32
  NonNegativeSignalChanged1 : PBCSimulinkLibrary/NonNegativeSignalChanged  SystemSampleTime=-1
  NonNegativeSignalChanged2 : PBCSimulinkLibrary/NonNegativeSignalChanged  SystemSampleTime=-1
  Bus : Outport
  wires:
  Double2Uint/1 -> Bus Creator1/2  "SPDIndex"
  NonNegativeSignalChanged2/1 -> Bus Creator1/3  "PowerDefined"
  NonNegativeSignalChanged1/1 -> Bus Creator1/1  "SPDIndexDefined"
  Power [W]/1 -> Bus Creator1/4, NonNegativeSignalChanged2/1  "Power"
  SPDIndex [-]/1 -> Double2Uint/1, NonNegativeSignalChanged1/1  "SPDIndex"
  Bus Creator1/1 -> Bus/1

== system Base_Map_S_P_L_cs/TrafficLightRoadSideNL_4/TrafficLightRoadSideNL_4_Casing.LightOrange_Control_Mux ==
  SPDIndex [-] : Inport
  Power [W] : Inport  Port=2
  Bus Creator1 : BusCreator  Inputs=4  OutDataTypeStr=Bus: PRESCAN_PBCLIGHT_DATA  NonVirtualBus=on
  Double2Uint : DataTypeConversion  OutDataTypeStr=uint32
  NonNegativeSignalChanged1 : PBCSimulinkLibrary/NonNegativeSignalChanged  SystemSampleTime=-1
  NonNegativeSignalChanged2 : PBCSimulinkLibrary/NonNegativeSignalChanged  SystemSampleTime=-1
  Bus : Outport
  wires:
  Double2Uint/1 -> Bus Creator1/2  "SPDIndex"
  NonNegativeSignalChanged2/1 -> Bus Creator1/3  "PowerDefined"
  NonNegativeSignalChanged1/1 -> Bus Creator1/1  "SPDIndexDefined"
  Power [W]/1 -> Bus Creator1/4, NonNegativeSignalChanged2/1  "Power"
  SPDIndex [-]/1 -> Double2Uint/1, NonNegativeSignalChanged1/1  "SPDIndex"
  Bus Creator1/1 -> Bus/1

== system Base_Map_S_P_L_cs/TrafficLightRoadSideNL_4/TrafficLightRoadSideNL_4_Casing.LightRed_Control_Mux ==
  SPDIndex [-] : Inport
  Power [W] : Inport  Port=2
  Bus Creator1 : BusCreator  Inputs=4  OutDataTypeStr=Bus: PRESCAN_PBCLIGHT_DATA  NonVirtualBus=on
  Double2Uint : DataTypeConversion  OutDataTypeStr=uint32
  NonNegativeSignalChanged1 : PBCSimulinkLibrary/NonNegativeSignalChanged  SystemSampleTime=-1
  NonNegativeSignalChanged2 : PBCSimulinkLibrary/NonNegativeSignalChanged  SystemSampleTime=-1
  Bus : Outport
  wires:
  Double2Uint/1 -> Bus Creator1/2  "SPDIndex"
  NonNegativeSignalChanged2/1 -> Bus Creator1/3  "PowerDefined"
  NonNegativeSignalChanged1/1 -> Bus Creator1/1  "SPDIndexDefined"
  Power [W]/1 -> Bus Creator1/4, NonNegativeSignalChanged2/1  "Power"
  SPDIndex [-]/1 -> Double2Uint/1, NonNegativeSignalChanged1/1  "SPDIndex"
  Bus Creator1/1 -> Bus/1

== system Base_Map_S_P_L_cs/TrafficLightRoadSideNL_4/VISUCasingLights_Mux ==
  Green [-] : Inport  Tag=inport/Green [-]  SampleTime=1/300  BusOutputAsStruct=on
  Orange [-] : Inport  Tag=inport/Orange [-]  Port=2  SampleTime=1/300  BusOutputAsStruct=on
  Red [-] : Inport  Tag=inport/Red [-]  Port=3  SampleTime=1/300  BusOutputAsStruct=on
  MuxVisuLights : Mux  Inputs=3
  VISUCasingLights_TrafficLightRoadSideNL_4 : Outport  Tag=outport/VisuCasingLights  SampleTime=1/300
  wires:
  MuxVisuLights/1 -> VISUCasingLights_TrafficLightRoadSideNL_4/1
  Green [-]/1 -> MuxVisuLights/1
  Orange [-]/1 -> MuxVisuLights/2
  Red [-]/1 -> MuxVisuLights/3

== system Base_Map_S_P_L_cs/TrafficLightRoadSideNL_5/TrafficLightRoadSideNL_5_Casing.LightGreen_Control_Mux ==
  SPDIndex [-] : Inport
  Power [W] : Inport  Port=2
  Bus Creator1 : BusCreator  Inputs=4  OutDataTypeStr=Bus: PRESCAN_PBCLIGHT_DATA  NonVirtualBus=on
  Double2Uint : DataTypeConversion  OutDataTypeStr=uint32
  NonNegativeSignalChanged1 : PBCSimulinkLibrary/NonNegativeSignalChanged  SystemSampleTime=-1
  NonNegativeSignalChanged2 : PBCSimulinkLibrary/NonNegativeSignalChanged  SystemSampleTime=-1
  Bus : Outport
  wires:
  Double2Uint/1 -> Bus Creator1/2  "SPDIndex"
  NonNegativeSignalChanged2/1 -> Bus Creator1/3  "PowerDefined"
  NonNegativeSignalChanged1/1 -> Bus Creator1/1  "SPDIndexDefined"
  Power [W]/1 -> Bus Creator1/4, NonNegativeSignalChanged2/1  "Power"
  SPDIndex [-]/1 -> Double2Uint/1, NonNegativeSignalChanged1/1  "SPDIndex"
  Bus Creator1/1 -> Bus/1

== system Base_Map_S_P_L_cs/TrafficLightRoadSideNL_5/TrafficLightRoadSideNL_5_Casing.LightOrange_Control_Mux ==
  SPDIndex [-] : Inport
  Power [W] : Inport  Port=2
  Bus Creator1 : BusCreator  Inputs=4  OutDataTypeStr=Bus: PRESCAN_PBCLIGHT_DATA  NonVirtualBus=on
  Double2Uint : DataTypeConversion  OutDataTypeStr=uint32
  NonNegativeSignalChanged1 : PBCSimulinkLibrary/NonNegativeSignalChanged  SystemSampleTime=-1
  NonNegativeSignalChanged2 : PBCSimulinkLibrary/NonNegativeSignalChanged  SystemSampleTime=-1
  Bus : Outport
  wires:
  Double2Uint/1 -> Bus Creator1/2  "SPDIndex"
  NonNegativeSignalChanged2/1 -> Bus Creator1/3  "PowerDefined"
  NonNegativeSignalChanged1/1 -> Bus Creator1/1  "SPDIndexDefined"
  Power [W]/1 -> Bus Creator1/4, NonNegativeSignalChanged2/1  "Power"
  SPDIndex [-]/1 -> Double2Uint/1, NonNegativeSignalChanged1/1  "SPDIndex"
  Bus Creator1/1 -> Bus/1

== system Base_Map_S_P_L_cs/TrafficLightRoadSideNL_5/TrafficLightRoadSideNL_5_Casing.LightRed_Control_Mux ==
  SPDIndex [-] : Inport
  Power [W] : Inport  Port=2
  Bus Creator1 : BusCreator  Inputs=4  OutDataTypeStr=Bus: PRESCAN_PBCLIGHT_DATA  NonVirtualBus=on
  Double2Uint : DataTypeConversion  OutDataTypeStr=uint32
  NonNegativeSignalChanged1 : PBCSimulinkLibrary/NonNegativeSignalChanged  SystemSampleTime=-1
  NonNegativeSignalChanged2 : PBCSimulinkLibrary/NonNegativeSignalChanged  SystemSampleTime=-1
  Bus : Outport
  wires:
  Double2Uint/1 -> Bus Creator1/2  "SPDIndex"
  NonNegativeSignalChanged2/1 -> Bus Creator1/3  "PowerDefined"
  NonNegativeSignalChanged1/1 -> Bus Creator1/1  "SPDIndexDefined"
  Power [W]/1 -> Bus Creator1/4, NonNegativeSignalChanged2/1  "Power"
  SPDIndex [-]/1 -> Double2Uint/1, NonNegativeSignalChanged1/1  "SPDIndex"
  Bus Creator1/1 -> Bus/1

== system Base_Map_S_P_L_cs/TrafficLightRoadSideNL_5/VISUCasingLights_Mux ==
  Green [-] : Inport  Tag=inport/Green [-]  SampleTime=1/300  BusOutputAsStruct=on
  Orange [-] : Inport  Tag=inport/Orange [-]  Port=2  SampleTime=1/300  BusOutputAsStruct=on
  Red [-] : Inport  Tag=inport/Red [-]  Port=3  SampleTime=1/300  BusOutputAsStruct=on
  MuxVisuLights : Mux  Inputs=3
  VISUCasingLights_TrafficLightRoadSideNL_5 : Outport  Tag=outport/VisuCasingLights  SampleTime=1/300
  wires:
  MuxVisuLights/1 -> VISUCasingLights_TrafficLightRoadSideNL_5/1
  Green [-]/1 -> MuxVisuLights/1
  Orange [-]/1 -> MuxVisuLights/2
  Red [-]/1 -> MuxVisuLights/3

== system Base_Map_S_P_L_cs/TrafficLightRoadSideNL_6/TrafficLightRoadSideNL_6_Casing.LightGreen_Control_Mux ==
  SPDIndex [-] : Inport
  Power [W] : Inport  Port=2
  Bus Creator1 : BusCreator  Inputs=4  OutDataTypeStr=Bus: PRESCAN_PBCLIGHT_DATA  NonVirtualBus=on
  Double2Uint : DataTypeConversion  OutDataTypeStr=uint32
  NonNegativeSignalChanged1 : PBCSimulinkLibrary/NonNegativeSignalChanged  SystemSampleTime=-1
  NonNegativeSignalChanged2 : PBCSimulinkLibrary/NonNegativeSignalChanged  SystemSampleTime=-1
  Bus : Outport
  wires:
  Double2Uint/1 -> Bus Creator1/2  "SPDIndex"
  NonNegativeSignalChanged2/1 -> Bus Creator1/3  "PowerDefined"
  NonNegativeSignalChanged1/1 -> Bus Creator1/1  "SPDIndexDefined"
  Power [W]/1 -> Bus Creator1/4, NonNegativeSignalChanged2/1  "Power"
  SPDIndex [-]/1 -> Double2Uint/1, NonNegativeSignalChanged1/1  "SPDIndex"
  Bus Creator1/1 -> Bus/1

== system Base_Map_S_P_L_cs/TrafficLightRoadSideNL_6/TrafficLightRoadSideNL_6_Casing.LightOrange_Control_Mux ==
  SPDIndex [-] : Inport
  Power [W] : Inport  Port=2
  Bus Creator1 : BusCreator  Inputs=4  OutDataTypeStr=Bus: PRESCAN_PBCLIGHT_DATA  NonVirtualBus=on
  Double2Uint : DataTypeConversion  OutDataTypeStr=uint32
  NonNegativeSignalChanged1 : PBCSimulinkLibrary/NonNegativeSignalChanged  SystemSampleTime=-1
  NonNegativeSignalChanged2 : PBCSimulinkLibrary/NonNegativeSignalChanged  SystemSampleTime=-1
  Bus : Outport
  wires:
  Double2Uint/1 -> Bus Creator1/2  "SPDIndex"
  NonNegativeSignalChanged2/1 -> Bus Creator1/3  "PowerDefined"
  NonNegativeSignalChanged1/1 -> Bus Creator1/1  "SPDIndexDefined"
  Power [W]/1 -> Bus Creator1/4, NonNegativeSignalChanged2/1  "Power"
  SPDIndex [-]/1 -> Double2Uint/1, NonNegativeSignalChanged1/1  "SPDIndex"
  Bus Creator1/1 -> Bus/1

== system Base_Map_S_P_L_cs/TrafficLightRoadSideNL_6/TrafficLightRoadSideNL_6_Casing.LightRed_Control_Mux ==
  SPDIndex [-] : Inport
  Power [W] : Inport  Port=2
  Bus Creator1 : BusCreator  Inputs=4  OutDataTypeStr=Bus: PRESCAN_PBCLIGHT_DATA  NonVirtualBus=on
  Double2Uint : DataTypeConversion  OutDataTypeStr=uint32
  NonNegativeSignalChanged1 : PBCSimulinkLibrary/NonNegativeSignalChanged  SystemSampleTime=-1
  NonNegativeSignalChanged2 : PBCSimulinkLibrary/NonNegativeSignalChanged  SystemSampleTime=-1
  Bus : Outport
  wires:
  Double2Uint/1 -> Bus Creator1/2  "SPDIndex"
  NonNegativeSignalChanged2/1 -> Bus Creator1/3  "PowerDefined"
  NonNegativeSignalChanged1/1 -> Bus Creator1/1  "SPDIndexDefined"
  Power [W]/1 -> Bus Creator1/4, NonNegativeSignalChanged2/1  "Power"
  SPDIndex [-]/1 -> Double2Uint/1, NonNegativeSignalChanged1/1  "SPDIndex"
  Bus Creator1/1 -> Bus/1

== system Base_Map_S_P_L_cs/TrafficLightRoadSideNL_6/VISUCasingLights_Mux ==
  Green [-] : Inport  Tag=inport/Green [-]  SampleTime=1/300  BusOutputAsStruct=on
  Orange [-] : Inport  Tag=inport/Orange [-]  Port=2  SampleTime=1/300  BusOutputAsStruct=on
  Red [-] : Inport  Tag=inport/Red [-]  Port=3  SampleTime=1/300  BusOutputAsStruct=on
  MuxVisuLights : Mux  Inputs=3
  VISUCasingLights_TrafficLightRoadSideNL_6 : Outport  Tag=outport/VisuCasingLights  SampleTime=1/300
  wires:
  MuxVisuLights/1 -> VISUCasingLights_TrafficLightRoadSideNL_6/1
  Green [-]/1 -> MuxVisuLights/1
  Orange [-]/1 -> MuxVisuLights/2
  Red [-]/1 -> MuxVisuLights/3

== system Base_Map_S_P_L_cs/TrafficLightRoadSideNL_7/TrafficLightRoadSideNL_7_Casing.LightGreen_Control_Mux ==
  SPDIndex [-] : Inport
  Power [W] : Inport  Port=2
  Bus Creator1 : BusCreator  Inputs=4  OutDataTypeStr=Bus: PRESCAN_PBCLIGHT_DATA  NonVirtualBus=on
  Double2Uint : DataTypeConversion  OutDataTypeStr=uint32
  NonNegativeSignalChanged1 : PBCSimulinkLibrary/NonNegativeSignalChanged  SystemSampleTime=-1
  NonNegativeSignalChanged2 : PBCSimulinkLibrary/NonNegativeSignalChanged  SystemSampleTime=-1
  Bus : Outport
  wires:
  Double2Uint/1 -> Bus Creator1/2  "SPDIndex"
  NonNegativeSignalChanged2/1 -> Bus Creator1/3  "PowerDefined"
  NonNegativeSignalChanged1/1 -> Bus Creator1/1  "SPDIndexDefined"
  Power [W]/1 -> Bus Creator1/4, NonNegativeSignalChanged2/1  "Power"
  SPDIndex [-]/1 -> Double2Uint/1, NonNegativeSignalChanged1/1  "SPDIndex"
  Bus Creator1/1 -> Bus/1

== system Base_Map_S_P_L_cs/TrafficLightRoadSideNL_7/TrafficLightRoadSideNL_7_Casing.LightOrange_Control_Mux ==
  SPDIndex [-] : Inport
  Power [W] : Inport  Port=2
  Bus Creator1 : BusCreator  Inputs=4  OutDataTypeStr=Bus: PRESCAN_PBCLIGHT_DATA  NonVirtualBus=on
  Double2Uint : DataTypeConversion  OutDataTypeStr=uint32
  NonNegativeSignalChanged1 : PBCSimulinkLibrary/NonNegativeSignalChanged  SystemSampleTime=-1
  NonNegativeSignalChanged2 : PBCSimulinkLibrary/NonNegativeSignalChanged  SystemSampleTime=-1
  Bus : Outport
  wires:
  Double2Uint/1 -> Bus Creator1/2  "SPDIndex"
  NonNegativeSignalChanged2/1 -> Bus Creator1/3  "PowerDefined"
  NonNegativeSignalChanged1/1 -> Bus Creator1/1  "SPDIndexDefined"
  Power [W]/1 -> Bus Creator1/4, NonNegativeSignalChanged2/1  "Power"
  SPDIndex [-]/1 -> Double2Uint/1, NonNegativeSignalChanged1/1  "SPDIndex"
  Bus Creator1/1 -> Bus/1

== system Base_Map_S_P_L_cs/TrafficLightRoadSideNL_7/TrafficLightRoadSideNL_7_Casing.LightRed_Control_Mux ==
  SPDIndex [-] : Inport
  Power [W] : Inport  Port=2
  Bus Creator1 : BusCreator  Inputs=4  OutDataTypeStr=Bus: PRESCAN_PBCLIGHT_DATA  NonVirtualBus=on
  Double2Uint : DataTypeConversion  OutDataTypeStr=uint32
  NonNegativeSignalChanged1 : PBCSimulinkLibrary/NonNegativeSignalChanged  SystemSampleTime=-1
  NonNegativeSignalChanged2 : PBCSimulinkLibrary/NonNegativeSignalChanged  SystemSampleTime=-1
  Bus : Outport
  wires:
  Double2Uint/1 -> Bus Creator1/2  "SPDIndex"
  NonNegativeSignalChanged2/1 -> Bus Creator1/3  "PowerDefined"
  NonNegativeSignalChanged1/1 -> Bus Creator1/1  "SPDIndexDefined"
  Power [W]/1 -> Bus Creator1/4, NonNegativeSignalChanged2/1  "Power"
  SPDIndex [-]/1 -> Double2Uint/1, NonNegativeSignalChanged1/1  "SPDIndex"
  Bus Creator1/1 -> Bus/1

== system Base_Map_S_P_L_cs/TrafficLightRoadSideNL_7/VISUCasingLights_Mux ==
  Green [-] : Inport  Tag=inport/Green [-]  SampleTime=1/300  BusOutputAsStruct=on
  Orange [-] : Inport  Tag=inport/Orange [-]  Port=2  SampleTime=1/300  BusOutputAsStruct=on
  Red [-] : Inport  Tag=inport/Red [-]  Port=3  SampleTime=1/300  BusOutputAsStruct=on
  MuxVisuLights : Mux  Inputs=3
  VISUCasingLights_TrafficLightRoadSideNL_7 : Outport  Tag=outport/VisuCasingLights  SampleTime=1/300
  wires:
  MuxVisuLights/1 -> VISUCasingLights_TrafficLightRoadSideNL_7/1
  Green [-]/1 -> MuxVisuLights/1
  Orange [-]/1 -> MuxVisuLights/2
  Red [-]/1 -> MuxVisuLights/3

== system Base_Map_S_P_L_cs/TrafficLightRoadSideNL_8/TrafficLightRoadSideNL_8_Casing.LightGreen_Control_Mux ==
  SPDIndex [-] : Inport
  Power [W] : Inport  Port=2
  Bus Creator1 : BusCreator  Inputs=4  OutDataTypeStr=Bus: PRESCAN_PBCLIGHT_DATA  NonVirtualBus=on
  Double2Uint : DataTypeConversion  OutDataTypeStr=uint32
  NonNegativeSignalChanged1 : PBCSimulinkLibrary/NonNegativeSignalChanged  SystemSampleTime=-1
  NonNegativeSignalChanged2 : PBCSimulinkLibrary/NonNegativeSignalChanged  SystemSampleTime=-1
  Bus : Outport
  wires:
  Double2Uint/1 -> Bus Creator1/2  "SPDIndex"
  NonNegativeSignalChanged2/1 -> Bus Creator1/3  "PowerDefined"
  NonNegativeSignalChanged1/1 -> Bus Creator1/1  "SPDIndexDefined"
  Power [W]/1 -> Bus Creator1/4, NonNegativeSignalChanged2/1  "Power"
  SPDIndex [-]/1 -> Double2Uint/1, NonNegativeSignalChanged1/1  "SPDIndex"
  Bus Creator1/1 -> Bus/1

== system Base_Map_S_P_L_cs/TrafficLightRoadSideNL_8/TrafficLightRoadSideNL_8_Casing.LightOrange_Control_Mux ==
  SPDIndex [-] : Inport
  Power [W] : Inport  Port=2
  Bus Creator1 : BusCreator  Inputs=4  OutDataTypeStr=Bus: PRESCAN_PBCLIGHT_DATA  NonVirtualBus=on
  Double2Uint : DataTypeConversion  OutDataTypeStr=uint32
  NonNegativeSignalChanged1 : PBCSimulinkLibrary/NonNegativeSignalChanged  SystemSampleTime=-1
  NonNegativeSignalChanged2 : PBCSimulinkLibrary/NonNegativeSignalChanged  SystemSampleTime=-1
  Bus : Outport
  wires:
  Double2Uint/1 -> Bus Creator1/2  "SPDIndex"
  NonNegativeSignalChanged2/1 -> Bus Creator1/3  "PowerDefined"
  NonNegativeSignalChanged1/1 -> Bus Creator1/1  "SPDIndexDefined"
  Power [W]/1 -> Bus Creator1/4, NonNegativeSignalChanged2/1  "Power"
  SPDIndex [-]/1 -> Double2Uint/1, NonNegativeSignalChanged1/1  "SPDIndex"
  Bus Creator1/1 -> Bus/1

== system Base_Map_S_P_L_cs/TrafficLightRoadSideNL_8/TrafficLightRoadSideNL_8_Casing.LightRed_Control_Mux ==
  SPDIndex [-] : Inport
  Power [W] : Inport  Port=2
  Bus Creator1 : BusCreator  Inputs=4  OutDataTypeStr=Bus: PRESCAN_PBCLIGHT_DATA  NonVirtualBus=on
  Double2Uint : DataTypeConversion  OutDataTypeStr=uint32
  NonNegativeSignalChanged1 : PBCSimulinkLibrary/NonNegativeSignalChanged  SystemSampleTime=-1
  NonNegativeSignalChanged2 : PBCSimulinkLibrary/NonNegativeSignalChanged  SystemSampleTime=-1
  Bus : Outport
  wires:
  Double2Uint/1 -> Bus Creator1/2  "SPDIndex"
  NonNegativeSignalChanged2/1 -> Bus Creator1/3  "PowerDefined"
  NonNegativeSignalChanged1/1 -> Bus Creator1/1  "SPDIndexDefined"
  Power [W]/1 -> Bus Creator1/4, NonNegativeSignalChanged2/1  "Power"
  SPDIndex [-]/1 -> Double2Uint/1, NonNegativeSignalChanged1/1  "SPDIndex"
  Bus Creator1/1 -> Bus/1

== system Base_Map_S_P_L_cs/TrafficLightRoadSideNL_8/VISUCasingLights_Mux ==
  Green [-] : Inport  Tag=inport/Green [-]  SampleTime=1/300  BusOutputAsStruct=on
  Orange [-] : Inport  Tag=inport/Orange [-]  Port=2  SampleTime=1/300  BusOutputAsStruct=on
  Red [-] : Inport  Tag=inport/Red [-]  Port=3  SampleTime=1/300  BusOutputAsStruct=on
  MuxVisuLights : Mux  Inputs=3
  VISUCasingLights_TrafficLightRoadSideNL_8 : Outport  Tag=outport/VisuCasingLights  SampleTime=1/300
  wires:
  MuxVisuLights/1 -> VISUCasingLights_TrafficLightRoadSideNL_8/1
  Green [-]/1 -> MuxVisuLights/1
  Orange [-]/1 -> MuxVisuLights/2
  Red [-]/1 -> MuxVisuLights/3

== system Base_Map_S_P_L_cs/VISUCasingLights_TrafficLightRoadSideNL_1/Actuator ==
  VISUCasingLights_TrafficLightRoadSideNL_1 : Inport  Tag=inport/VisuCasingLights  SampleTime=1/300  BusOutputAsStruct=on
  DemuxVisuLights : Demux  Outputs=3
  LimiterVisuLights : Saturate  UpperLimit=1  LowerLimit=0
  visu_Green [-] : S-Function  FunctionName=sfun_MaterialColorSelector  Parameters=mbxruntime.parameters.convert(UniqueID), mbxruntime.parameters.convert(ColorsObjectQuery), mbxruntime.parameters.convert(Colors),tabledata, TimeStep  SFunctionDeploymentMode=off  EnableBusSupport=off  mask(PreScan Sink Block: VisuTrafficLight){UniqueID=646, ColorsObjectQuery=child:name=TrafficLightRoadSideNL_1.Casing.LightGreen, Colors=[5   32   25  255    0   64   50  255    0   64   50  255    0    0    0  255; 0   45   34  255    0   45   34  255    0   45   34  255   30  306  240  255], TimeStep=1/300}
      mask prompts: UniqueID "Parent Unique Identifier"; ColorsObjectQuery "Query for Color Object"; Colors "Matrix of colors"; TimeStep "Simulink time step"
      mask help:
      | The VisuTrafficLight block provides a way to animate traffic lights: switch on and off individual lights.
      |
      | For more information, please click Help.
      mask init:
      | [tabledata] = mbxruntime.parameters.table(UniqueID,ColorsObjectQuery,Colors);
      mask Help: eval('openHelp(731)')
      mask Display: image(imread('TrafficLightCasing.png'))
  visu_Orange [-] : S-Function  FunctionName=sfun_MaterialColorSelector  Parameters=mbxruntime.parameters.convert(UniqueID), mbxruntime.parameters.convert(ColorsObjectQuery), mbxruntime.parameters.convert(Colors),tabledata, TimeStep  SFunctionDeploymentMode=off  EnableBusSupport=off  mask(PreScan Sink Block: VisuTrafficLight){UniqueID=646, ColorsObjectQuery=child:name=TrafficLightRoadSideNL_1.Casing.LightOrange, Colors=[32   25    5  255   64   48    5  255   64   54    5  255    0    0    0  255; 45   34    0  255   45   34    0  255   45   34    0  255  306  229    5  255], TimeStep=1/300}
      mask prompts: UniqueID "Parent Unique Identifier"; ColorsObjectQuery "Query for Color Object"; Colors "Matrix of colors"; TimeStep "Simulink time step"
      mask help:
      | The VisuTrafficLight block provides a way to animate traffic lights: switch on and off individual lights.
      |
      | For more information, please click Help.
      mask init:
      | [tabledata] = mbxruntime.parameters.table(UniqueID,ColorsObjectQuery,Colors);
      mask Help: eval('openHelp(731)')
      mask Display: image(imread('TrafficLightCasing.png'))
  visu_Red [-] : S-Function  FunctionName=sfun_MaterialColorSelector  Parameters=mbxruntime.parameters.convert(UniqueID), mbxruntime.parameters.convert(ColorsObjectQuery), mbxruntime.parameters.convert(Colors),tabledata, TimeStep  SFunctionDeploymentMode=off  EnableBusSupport=off  mask(PreScan Sink Block: VisuTrafficLight){UniqueID=646, ColorsObjectQuery=child:name=TrafficLightRoadSideNL_1.Casing.LightRed, Colors=[32    5    5  255   64    5    5  255   64    5    5  255    0    0    0  255; 45    0    0  255   45    0    0  255   45    0    0  255  306   30   30  255], TimeStep=1/300}
      mask prompts: UniqueID "Parent Unique Identifier"; ColorsObjectQuery "Query for Color Object"; Colors "Matrix of colors"; TimeStep "Simulink time step"
      mask help:
      | The VisuTrafficLight block provides a way to animate traffic lights: switch on and off individual lights.
      |
      | For more information, please click Help.
      mask init:
      | [tabledata] = mbxruntime.parameters.table(UniqueID,ColorsObjectQuery,Colors);
      mask Help: eval('openHelp(731)')
      mask Display: image(imread('TrafficLightCasing.png'))
  wires:
  VISUCasingLights_TrafficLightRoadSideNL_1/1 -> LimiterVisuLights/1
  LimiterVisuLights/1 -> DemuxVisuLights/1
  DemuxVisuLights/1 -> visu_Green [-]/1
  DemuxVisuLights/2 -> visu_Orange [-]/1
  DemuxVisuLights/3 -> visu_Red [-]/1
